simulink model "SS_Harness"  (R2022b)
settings: configuration reference "CommonModelConfiguration" (kept outside this file)
(part 1 of 2)
settings Model: DataTypeOverride=Off  Creator=lcartea  LastModifiedBy=AJOSHI11
settings ConfigSetRef: SourceName=CommonModelConfiguration  SourceLocation=Base Workspace

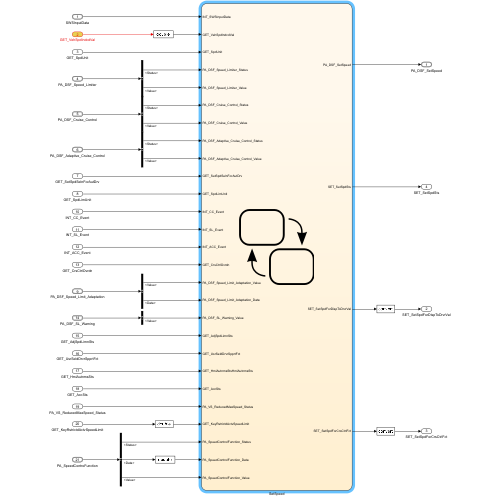
[thumbnail: Simulink's stored preview of the top-level diagram]
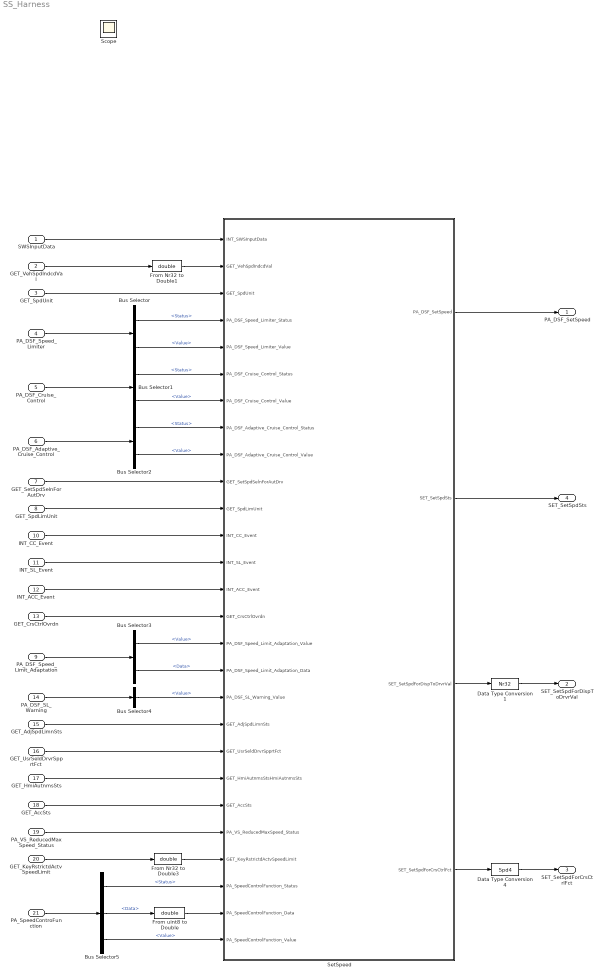
== system SS_Harness ==
  SWSInputData : Inport  OutDataTypeStr=Bus: SWSInputData  BusOutputAsStruct=on
  GET_VehSpdIndcdVal : Inport  Port=2  OutDataTypeStr=Nr32
  GET_SpdUnit : Inport  Port=3  OutDataTypeStr=Enum: VehSpdIndcdUnit
  PA_DSF_Speed_Limiter : Inport  Port=4  OutDataTypeStr=Bus: PA_DSF
  PA_DSF_Cruise_Control : Inport  Port=5  OutDataTypeStr=Bus: PA_DSF
  PA_DSF_Adaptive_Cruise_Control : Inport  Port=6  OutDataTypeStr=Bus: PA_DSF_ACC
  GET_SetSpdSelnForAutDrv : Inport  Port=7  OutDataTypeStr=Enum: SetSpdSelnForAutDrv1
  GET_SpdLimUnit : Inport  Port=8  OutDataTypeStr=Enum: SpdUnit1
  PA_DSF_Speed_Limit_Adaptation : Inport  Port=9  OutDataTypeStr=Bus: PA_DSF_SLA
  INT_CC_Event : Inport  Port=10  OutDataTypeStr=Enum: E_DSF_Event
  INT_SL_Event : Inport  Port=11  OutDataTypeStr=Enum: E_DSF_Event
  INT_ACC_Event : Inport  Port=12  OutDataTypeStr=Enum: E_DSF_Event
  GET_CrsCtrlOvrdn : Inport  Port=13  OutDataTypeStr=Enum: OnOff1
  PA_DSF_SL_Warning : Inport  Port=14  OutDataTypeStr=Bus: PA_StatusAndOffOnValue
  GET_AdjSpdLimnSts : Inport  Port=15  OutDataTypeStr=Enum: AdjSpdLimnSts2
  GET_UsrSeldDrvrSpprtFct : Inport  Port=16  OutDataTypeStr=Enum: DrvrSpprtFct
  GET_HmiAutnmsSts : Inport  Port=17  OutDataTypeStr=Enum: HmiAutnmsSts1
  GET_AccSts : Inport  Port=18  OutDataTypeStr=Enum: AccSts1
  PA_VS_ReducedMaxSpeed_Status : Inport  Port=19  OutDataTypeStr=Enum: E_CommonStatus
  GET_KeyRstrictdActvSpeedLimit : Inport  Port=20  OutDataTypeStr=Spd4
  PA_SpeedControFunction : Inport  Port=21  OutDataTypeStr=Bus: PA_StatusAnduIntAndOffOnValue
  Bus Selector : BusSelector  OutputSignals=Status,Value
  Bus Selector1 : BusSelector  OutputSignals=Status,Value
  Bus Selector2 : BusSelector  OutputSignals=Status,Value
  Bus Selector3 : BusSelector  OutputSignals=Value,Data
  Bus Selector4 : BusSelector  OutputSignals=Value
  Bus Selector5 : BusSelector  OutputSignals=Status,Data,Value
  Data Type Conversion1 : DataTypeConversion  OutDataTypeStr=Nr32  RndMeth=Round  SaturateOnIntegerOverflow=off
  Data Type Conversion4 : DataTypeConversion  OutDataTypeStr=Spd4  RndMeth=Round  SaturateOnIntegerOverflow=off
  From Nr32 to Double1 : DataTypeConversion  OutDataTypeStr=double  SaturateOnIntegerOverflow=off  RndMeth=Floor  LockScale=on
  From Nr32 to Double3 : DataTypeConversion  OutDataTypeStr=double  SaturateOnIntegerOverflow=off  RndMeth=Floor  LockScale=on
  From uint8 to Double : DataTypeConversion  OutDataTypeStr=double  SaturateOnIntegerOverflow=off  RndMeth=Floor
  SetSpeed : Stateflow chart  TreatAsAtomicUnit=on
  PA_DSF_SetSpeed : Outport  OutDataTypeStr=Bus: PA_StatusAndValueAndDoubleAndDouble  VectorParamsAs1DForOutWhenUnconnected=off  BusOutputAsStruct=on
  SET_SetSpdForDispToDrvrVal : Outport  Port=2  OutDataTypeStr=Nr32  VectorParamsAs1DForOutWhenUnconnected=off
  SET_SetSpdForCrsCtrlFct : Outport  Port=3  OutDataTypeStr=Spd4  VectorParamsAs1DForOutWhenUnconnected=off
  SET_SetSpdSts : Outport  Port=4  OutDataTypeStr=Enum: SetSpdSts1  VectorParamsAs1DForOutWhenUnconnected=off
  Scope : Scope
  wires:
  SWSInputData/1 -> SetSpeed/1(INT_SWSInputData)
  SetSpeed/3(SET_SetSpdForDispToDrvrVal) -> Data Type Conversion1/1
  GET_VehSpdIndcdVal/1 -> From Nr32 to Double1/1
  GET_SpdUnit/1 -> SetSpeed/3(GET_SpdUnit)
  PA_DSF_Speed_Limiter/1 -> Bus Selector/1
  PA_DSF_Cruise_Control/1 -> Bus Selector1/1
  PA_DSF_Adaptive_Cruise_Control/1 -> Bus Selector2/1
  From Nr32 to Double1/1 -> SetSpeed/2(GET_VehSpdIndcdVal)
  Data Type Conversion1/1 -> SET_SetSpdForDispToDrvrVal/1
  Bus Selector/1 -> SetSpeed/4(PA_DSF_Speed_Limiter_Status)  "<Status>"
  Bus Selector1/1 -> SetSpeed/6(PA_DSF_Cruise_Control_Status)  "<Status>"
  Bus Selector2/1 -> SetSpeed/8(PA_DSF_Adaptive_Cruise_Control_Status)  "<Status>"
  GET_SetSpdSelnForAutDrv/1 -> SetSpeed/10(GET_SetSpdSelnForAutDrv)
  GET_SpdLimUnit/1 -> SetSpeed/11(GET_SpdLimUnit)
  INT_CC_Event/1 -> SetSpeed/12(INT_CC_Event)
  INT_SL_Event/1 -> SetSpeed/13(INT_SL_Event)
  INT_ACC_Event/1 -> SetSpeed/14(INT_ACC_Event)
  SetSpeed/4(SET_SetSpdForCrsCtrlFct) -> Data Type Conversion4/1
  GET_CrsCtrlOvrdn/1 -> SetSpeed/15(GET_CrsCtrlOvrdn)
  Bus Selector2/2 -> SetSpeed/9(PA_DSF_Adaptive_Cruise_Control_Value)  "<Value>"
  PA_DSF_Speed_Limit_Adaptation/1 -> Bus Selector3/1
  Bus Selector3/1 -> SetSpeed/16(PA_DSF_Speed_Limit_Adaptation_Value)  "<Value>"
  Bus Selector3/2 -> SetSpeed/17(PA_DSF_Speed_Limit_Adaptation_Data)  "<Data>"
  Data Type Conversion4/1 -> SET_SetSpdForCrsCtrlFct/1
  SetSpeed/1(PA_DSF_SetSpeed) -> PA_DSF_SetSpeed/1
  PA_DSF_SL_Warning/1 -> Bus Selector4/1
  GET_AdjSpdLimnSts/1 -> SetSpeed/19(GET_AdjSpdLimnSts)
  Bus Selector4/1 -> SetSpeed/18(PA_DSF_SL_Warning_Value)  "<Value>"
  GET_UsrSeldDrvrSpprtFct/1 -> SetSpeed/20(GET_UsrSeldDrvrSpprtFct)
  GET_HmiAutnmsSts/1 -> SetSpeed/21(GET_HmiAutnmsStsHmiAutnmsSts)
  GET_AccSts/1 -> SetSpeed/22(GET_AccSts)
  Bus Selector/2 -> SetSpeed/5(PA_DSF_Speed_Limiter_Value)  "<Value>"
  Bus Selector1/2 -> SetSpeed/7(PA_DSF_Cruise_Control_Value)  "<Value>"
  GET_KeyRstrictdActvSpeedLimit/1 -> From Nr32 to Double3/1
  From Nr32 to Double3/1 -> SetSpeed/24(GET_KeyRstrictdActvSpeedLimit)
  PA_VS_ReducedMaxSpeed_Status/1 -> SetSpeed/23(PA_VS_ReducedMaxSpeed_Status)
  PA_SpeedControFunction/1 -> Bus Selector5/1
  Bus Selector5/1 -> SetSpeed/25(PA_SpeedControlFunction_Status)  "<Status>"
  Bus Selector5/3 -> SetSpeed/27(PA_SpeedControlFunction_Value)  "<Value>"
  Bus Selector5/2 -> From uint8 to Double/1  "<Data>"
  From uint8 to Double/1 -> SetSpeed/26(PA_SpeedControlFunction_Data)
  SetSpeed/2(SET_SetSpdSts) -> SET_SetSpdSts/1
